simulink model "sensorless_MRAS_pmsm"  (Simulink 7.6)
settings: Solver=ode23tb  StartTime=0.0  StopTime=0.4  RelTol=1e-3
libraries: powerlib x11
settings Model: Creator=1  LastModifiedBy=1
settings OptimizationCC: InitFltsAndDblsToZero=on
settings DebuggingCC: SaveWithParameterizedLinksMsg=none  SignalResolutionControl=TryResolveAllWithWarning  MultiTaskDSMMsg=warning  MultiTaskCondExecSysMsg=none  UnconnectedLineMsg=none  StrictBusMsg=Warning
settings RTWCC: IncludeERTFirstTime=on
settings GRTTargetCC: TargetFcnLib=ansi_tfl_tmw.mat

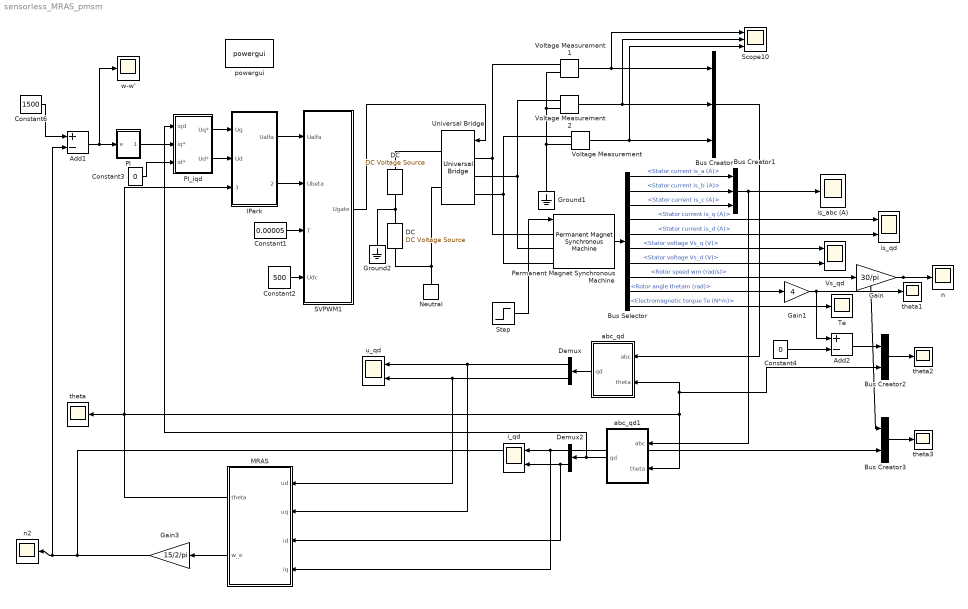
== system sensorless_MRAS_pmsm ==
  Add1 : Sum  Inputs=+-
  Add2 : Sum  Inputs=+-
  Bus Creator : BusCreator  Inputs=3
  Bus Creator1 : BusCreator  Inputs=3
  Bus Creator2 : BusCreator  Inputs=2
  Bus Creator3 : BusCreator  Inputs=2
  Bus Selector : BusSelector  OutputSignals=Stator current is_a (A),Stator current is_b (A),Stator current is_c (A),Stator current is_q (A),Stator current is_d (A),Stator voltage Vs_q (V),Stator voltage Vs_d (V),Rotor speed wm (rad/s),Rotor angle thetam (rad),Electromagnetic torque Te (N*m)
  Constant1 : Constant  Value=0.00005
  Constant2 : Constant  Value=500
  Constant3 : Constant  Value=0
  Constant4 : Constant  Value=0
  Constant6 : Constant  Value=1500
  DC : powerlib/Electrical Sources/DC Voltage Source  DialogController=POWERSYS.PowerSysDialog  SystemSampleTime=-1  Amplitude=250  Measurements=None
  "DC " : powerlib/Electrical Sources/DC Voltage Source  DialogController=POWERSYS.PowerSysDialog  SystemSampleTime=-1  Amplitude=250  Measurements=None
  Demux : Demux  Outputs=2
  Demux2 : Demux  Outputs=2
  Gain : Gain  Gain=30/pi
  Gain1 : Gain  Gain=4
  Gain3 : Gain  Gain=15/2/pi
  Ground1 : powerlib/Elements/Ground  DialogController=POWERSYS.PowerSysDialog  PhysicalDomain=powersysdomain  SubClassName=unknown  LeftPortType=p1  RightPortType=p1  LConnTagsString=a
  Ground2 : powerlib/Elements/Ground  DialogController=POWERSYS.PowerSysDialog  PhysicalDomain=powersysdomain  SubClassName=unknown  LeftPortType=p1  RightPortType=p1  LConnTagsString=a
  IPark : Subsystem
  MRAS : Subsystem
  Neutral : powerlib/Elements/Neutral  DialogController=POWERSYS.PowerSysDialog  PhysicalDomain=powersysdomain  SubClassName=unknown  LeftPortType=p1  RightPortType=p1  LConnTagsString=a  NodeNumber=10
  PI : Subsystem
  PI_iqd : Subsystem
  Permanent Magnet Synchronous Machine : powerlib/Machines/Permanent Magnet Synchronous Machine  DialogController=POWERSYS.PowerSysDialog  SystemSampleTime=-1  FluxDistribution=Sinusoidal  MechanicalLoad=Torque Tm  PresetModel=No  ShowDetailedParameters=on  Resistance=2.8750  Inductance=8.5e-3  dqInductances=[8.5e-3, 8.5e-3]  MachineConstant=Flux linkage established by magnets (V.s)  Flux=0.175  VoltageCst=126.966  TorqueCst=1.05  Flat=120  Mechanical="[ 1e-3, 0,  4 ]"  PolePairs=4  InitialConditions=[0,0, 0,0]  TsPowergui=0  TsBlock=-1
  SVPWM1 : Subsystem
  Scope10 : Scope  NumInputPorts=3
      settings: TimeRange=0.2  YMin=-250~-250~-250  YMax=250~250~250  SaveName=ScopeData22  DataFormat=Structure
  Step : Step  Time=0.2  SampleTime=0
  Te : Scope
      settings: YMin=1.775  YMax=2.225  SaveName=ScopeData6
  Universal Bridge : powerlib/Power Electronics/Universal Bridge  DialogController=POWERSYS.PowerSysDialog  SystemSampleTime=-1  Arms=3  SnubberResistance=1e5  SnubberCapacitance=inf  Device=IGBT / Diodes  Ron=1e-3  Lon=0  ForwardVoltages="[  0  0  ]"  ForwardVoltage=0  GTOparameters=[ 10e-6 , 20e-6 ]  IGBTparameters=[ 1e-6 , 2e-6 ]  Measurements=None  Measurements_2=None  converterType=Rectifier
  Voltage Measurement : powerlib/Measurements/Voltage Measurement  DialogController=POWERSYS.PowerSysDialog  SystemSampleTime=-1  PhasorSimulation=off  OutputType=Complex  PSBequivalent=0
  Voltage Measurement1 : powerlib/Measurements/Voltage Measurement  DialogController=POWERSYS.PowerSysDialog  SystemSampleTime=-1  PhasorSimulation=off  OutputType=Complex  PSBequivalent=0
  Voltage Measurement2 : powerlib/Measurements/Voltage Measurement  DialogController=POWERSYS.PowerSysDialog  SystemSampleTime=-1  PhasorSimulation=off  OutputType=Complex  PSBequivalent=0
  Vs_qd : Scope  NumInputPorts=2
      settings: TimeRange=0.4  YMin=-400~-99.99999999999994  YMax=400~-67.44186046511635  SaveName=ScopeData8
  abc_qd : Subsystem
  abc_qd1 : Subsystem
  "i_qd " : Scope  NumInputPorts=2
      settings: TimeRange=0.06  YMin=1.675~-0.475  YMax=2.075~-0.225  SaveName=ScopeData27  DataFormat=Structure
  is_abc (A) : Scope
      settings: TimeRange=0.06  YMin=-1.5  YMax=1.25  DataFormat=Structure
  is_qd : Scope  NumInputPorts=2
      settings: TimeRange=0.2  YMin=1.7~-0.23  YMax=2.1~-0.04  SaveName=ScopeData4
  n : Scope
      settings: TimeRange=0.0005809128630705485  YMin=2064.7  YMax=2065.35  SaveName=ScopeData15
  n2 : Scope
      settings: YMin=1470  YMax=1530  SaveName=ScopeData18
  powergui : powerlib/powergui  Priority=1  SystemSampleTime=-1  SimulationMode=Continuous  SampleTime=50e-6  frequency=60  SPID=off  DisableSnubberDevices=off  DisableRonSwitches=off  DisableVfSwitches=off  SwTol=0  Interpol=off  frequencyindice=0  echomessages=off  HookPort=off  DisplayEquations=off  FunctionMessages=off  EnableUseOfTLC=off  x0status=blocks  RestoreLinks=warning  ResistiveCurrentMeasurement=off  Ylog=off  Xlog=on  ShowGrid=off  save=off  variable=ZData  ZoomFFT=off  StartTime=0.0  cycles=1  DisplayStyle=1  FreqAxis=off  MaxFrequency=1000  frequencyindicesteady=1  display=off  methode=off
  theta{,1..3} (4 alike) : Scope
      theta settings: YMin=67.3  YMax=68.15  SaveName=ScopeData17
      theta1 settings: TimeRange=0.2  YMin=-3.955  YMax=-3.88  SaveName=ScopeData5
      theta2 settings: TimeRange=0.2  YMin=-10  YMax=55  SaveName=ScopeData7
      theta3 settings: TimeRange=0.2  YMin=-3.955  YMax=-3.88  SaveName=ScopeData14
  "u_qd " : Scope  NumInputPorts=2
      settings: TimeRange=0.06  YMin=-25~-250  YMax=325~350  SaveName=ScopeData26  DataFormat=Structure
  w-w' : Scope
      settings: TimeRange=0.02  YMin=-6  YMax=6  SaveName=ScopeData3
  wires:
  Constant3/1 -> PI_iqd/3(id*)
  Constant2/1 -> SVPWM1/4(Udc)
  Constant1/1 -> SVPWM1/3(T)
  Add1/1 -> PI/1(e), w-w'/1
  Constant6/1 -> Add1/1
  SVPWM1/1(Ugate) -> Universal Bridge/1
  IPark/1(Ualfa) -> SVPWM1/1(Ualfa)
  IPark/2(Ubeta) -> SVPWM1/2(Ubeta)
  Voltage Measurement/1 -> Scope10/3, Bus Creator/3
  Voltage Measurement2/1 -> Scope10/2, Bus Creator/2
  Voltage Measurement1/1 -> Scope10/1, Bus Creator/1
  Demux/1 -> "u_qd "/1, MRAS/2(uq)
  Demux/2 -> "u_qd "/2, MRAS/1(ud)
  Demux2/1 -> "i_qd "/1, MRAS/4(iq)
  Demux2/2 -> "i_qd "/2, MRAS/3(id)
  PI_iqd/2(Ud*) -> IPark/2(Ud)
  PI_iqd/1(Uq*) -> IPark/1(Uq)
  Permanent Magnet Synchronous Machine/1 -> Bus Selector/1
  Bus Selector/1 -> Bus Creator1/1  "<Stator current is_a (A)>"
  Bus Selector/2 -> Bus Creator1/2  "<Stator current is_b (A)>"
  Bus Selector/3 -> Bus Creator1/3  "<Stator current is_c (A)>"
  Bus Selector/4 -> is_qd/1  "<Stator current is_q (A)>"
  Bus Selector/5 -> is_qd/2  "<Stator current is_d (A)>"
  Bus Selector/6 -> Vs_qd/1  "<Stator voltage Vs_q (V)>"
  Bus Selector/7 -> Vs_qd/2  "<Stator voltage Vs_d (V)>"
  Gain/1 -> n/1, Bus Creator3/1
  Bus Selector/8 -> Gain/1  "<Rotor speed wm (rad/s)>"
  Bus Selector/9 -> Gain1/1  "<Rotor angle thetam (rad)>"
  Gain1/1 -> theta1/1, Add2/1
  Bus Selector/10 -> Te/1  "<Electromagnetic torque Te (N*m)>"
  Bus Creator1/1 -> is_abc (A)/1, abc_qd1/1(abc)
  Step/1 -> Permanent Magnet Synchronous Machine/1
  abc_qd/1(qd) -> Demux/1
  Gain3/1 -> n2/1, Add1/2, Bus Creator3/2
  abc_qd1/1(qd) -> Demux2/1, PI_iqd/1(iqd)
  MRAS/1(theta) -> IPark/3(thetma), abc_qd1/2(theta), abc_qd/2(theta), Bus Creator2/2, theta/1
  Bus Creator/1 -> abc_qd/1(abc)
  MRAS/2(w_e) -> Gain3/1
  PI/1(iq*) -> PI_iqd/2(iq*)
  Bus Creator2/1 -> theta2/1
  Bus Creator3/1 -> theta3/1
  Add2/1 -> Bus Creator2/1
  Constant4/1 -> Add2/2
  connections:
  Universal Bridge/RConn1 -- "DC "/RConn1
  DC/RConn1 -- "DC "/LConn1 -- Ground2/LConn1
  Voltage Measurement1/LConn2 -- Voltage Measurement2/LConn2 -- Ground1/LConn1 -- Voltage Measurement/LConn2
  DC/LConn1 -- Universal Bridge/RConn2 -- Neutral/LConn1
  Permanent Magnet Synchronous Machine/LConn1 -- Universal Bridge/LConn1 -- Voltage Measurement1/LConn1
  Permanent Magnet Synchronous Machine/LConn2 -- Universal Bridge/LConn2 -- Voltage Measurement2/LConn1
  Permanent Magnet Synchronous Machine/LConn3 -- Universal Bridge/LConn3 -- Voltage Measurement/LConn1

== system sensorless_MRAS_pmsm/IPark ==
  Uq : Inport
  Ud : Inport  Port=2
  thetma : Inport  Port=3
  Fcn : Fcn  Expr=cos(u[3])*u[2]-sin(u[3])*u[1]
  Fcn1 : Fcn  Expr=sin(u[3])*u[2]+cos(u[3])*u[1]
  Mux : Mux  Inputs=3
  Scope6 : Scope  NumInputPorts=2
      settings: YMin=40~20  YMax=230~220  SaveName=ScopeData12
  Ualfa : Outport
  Ubeta : Outport  Port=2
  wires:
  Uq/1 -> Mux/1
  Ud/1 -> Mux/2
  thetma/1 -> Mux/3
  Mux/1 -> Fcn/1, Fcn1/1
  Fcn/1 -> Ualfa/1, Scope6/1
  Fcn1/1 -> Ubeta/1, Scope6/2

== system sensorless_MRAS_pmsm/MRAS ==
  ud : Inport
  uq : Inport  Port=2
  id : Inport  Port=3
  iq : Inport  Port=4
  Integrator : Integrator
  Iqd : Subsystem
  "i_qd " : Scope  NumInputPorts=2
      settings: TimeRange=0.06  YMin=-4~0.5  YMax=16~10  SaveName=ScopeData23  DataFormat=Structure
  i_qd 1 : Scope  NumInputPorts=2
      settings: TimeRange=0.06  YMin=3.375~-1.525  YMax=3.8~-1.275  SaveName=ScopeData28  DataFormat=Structure
  we : Subsystem
  theta : Outport
  w_e : Outport  Port=2
  wires:
  ud/1 -> Iqd/1(ud)
  uq/1 -> Iqd/2(uq)
  iq/1 -> we/2(iq), "i_qd "/1
  Iqd/1(i_d) -> i_qd 1/2, we/3(i_d)
  Iqd/2(i_q) -> we/4(i_q), i_qd 1/1
  we/1(w_e) -> Integrator/1, w_e/1, Iqd/3(we)
  Integrator/1 -> theta/1
  id/1 -> we/1(id), "i_qd "/2

== system sensorless_MRAS_pmsm/PI ==
  e : Inport
  Integrator : Integrator
  Ks : Gain
  Ks/ts : Gain  Gain=0.02
  Saturation : Saturate  UpperLimit=21  LowerLimit=-21
  Sum1 : Sum  Inputs=|++
  iq* : Outport
  wires:
  Ks/1 -> Sum1/1
  Ks/ts/1 -> Integrator/1
  Integrator/1 -> Sum1/2
  e/1 -> Ks/1, Ks/ts/1
  Sum1/1 -> Saturation/1
  Saturation/1 -> iq*/1

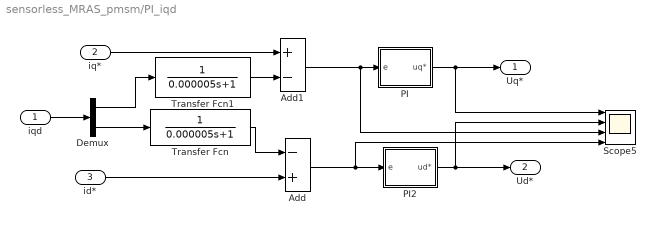
== system sensorless_MRAS_pmsm/PI_iqd ==
  iqd : Inport
  iq* : Inport  Port=2
  id* : Inport  Port=3
  Add : Sum  Inputs=-+
  Add1 : Sum  Inputs=+-
  Demux : Demux  Outputs=2
  PI : Subsystem
  PI2 : Subsystem
  Scope5 : Scope  NumInputPorts=4
      settings: YMin=218.5~-9.25~-0.2~-0.04  YMax=225~-7.75~0.25~0.06  SaveName=ScopeData10
  Transfer Fcn : TransferFcn  Denominator=[0.000005 1]
  Transfer Fcn1 : TransferFcn  Denominator=[0.000005 1]
  Uq* : Outport
  Ud* : Outport  Port=2
  wires:
  iqd/1 -> Demux/1
  id*/1 -> Add/2
  Add1/1 -> PI/1(e), Scope5/3
  Add/1 -> PI2/1(e), Scope5/4
  PI2/1(ud*) -> Ud*/1, Scope5/2
  PI/1(uq*) -> Uq*/1, Scope5/1
  Demux/1 -> Transfer Fcn1/1
  Transfer Fcn1/1 -> Add1/2
  Demux/2 -> Transfer Fcn/1
  Transfer Fcn/1 -> Add/1
  iq*/1 -> Add1/1

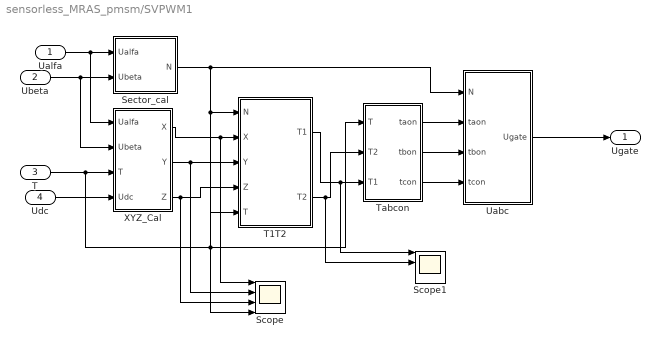
== system sensorless_MRAS_pmsm/SVPWM1 ==
  Ualfa : Inport
  Ubeta : Inport  Port=2
  T : Inport  Port=3
  Udc : Inport  Port=4
  Scope : Scope  NumInputPorts=4
      settings: YMin=0~-0.00015~1e-005~4.75  YMax=1.1e-020~-1e-005~0.00015~5.25  SaveName=ScopeData2
  Scope1 : Scope  NumInputPorts=4
      settings: YMin=3e-006~6.61744e-024~1e-005~4.75  YMax=1.6e-005~1e-007~0.00015~5.25  SaveName=ScopeData13
  Sector_cal : Subsystem
  T1T2 : Subsystem
  Tabcon : Subsystem
  Uabc : Subsystem
  XYZ_Cal : Subsystem
  Ugate : Outport
  wires:
  Sector_cal/1(N) -> Uabc/1(N), T1T2/1(N), Scope/4
  Ualfa/1 -> XYZ_Cal/1(Ualfa), Sector_cal/1(Ualfa)
  Ubeta/1 -> XYZ_Cal/2(Ubeta), Sector_cal/2(Ubeta)
  T/1 -> XYZ_Cal/3(T), Tabcon/1(T), T1T2/5(T)
  Udc/1 -> XYZ_Cal/4(Udc)
  XYZ_Cal/1(X) -> T1T2/2(X), Scope/1
  XYZ_Cal/2(Y) -> T1T2/3(Y), Scope/2
  XYZ_Cal/3(Z) -> T1T2/4(Z), Scope/3
  T1T2/2(T2) -> Tabcon/2(T2), Scope1/2
  T1T2/1(T1) -> Tabcon/3(T1), Scope1/1
  Tabcon/1(taon) -> Uabc/2(taon)
  Tabcon/2(tbon) -> Uabc/3(tbon)
  Tabcon/3(tcon) -> Uabc/4(tcon)
  Uabc/1(Ugate) -> Ugate/1

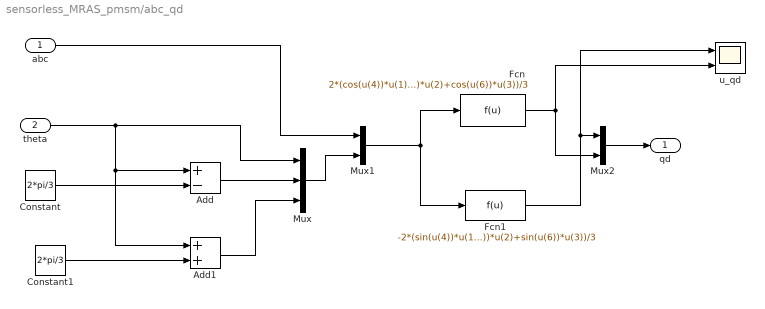
== system sensorless_MRAS_pmsm/abc_qd ==
  abc : Inport
  theta : Inport  Port=2
  Add : Sum  Inputs=+-
  Add1 : Sum
  Constant : Constant  Value=2*pi/3
  Constant1 : Constant  Value=2*pi/3
  Fcn : Fcn  Expr=2*(cos(u(4))*u(1)+cos(u(5))*u(2)+cos(u(6))*u(3))/3
  Fcn1 : Fcn  Expr=-2*(sin(u(4))*u(1)+sin(u(5))*u(2)+sin(u(6))*u(3))/3
  Mux : Mux  Inputs=3
  Mux1 : Mux  Inputs=2
  Mux2 : Mux  Inputs=2
  "u_qd " : Scope  NumInputPorts=2
      settings: TimeRange=0.06  YMin=-25~-300  YMax=300~250  SaveName=ScopeData24  DataFormat=Structure
  qd : Outport
  wires:
  Constant1/1 -> Add1/2
  Constant/1 -> Add/2
  theta/1 -> Mux/1, Add1/1, Add/1
  Add/1 -> Mux/2
  Add1/1 -> Mux/3
  Mux/1 -> Mux1/2
  abc/1 -> Mux1/1
  Mux1/1 -> Fcn/1, Fcn1/1
  Mux2/1 -> qd/1
  Fcn/1 -> Mux2/2, "u_qd "/2
  Fcn1/1 -> Mux2/1, "u_qd "/1

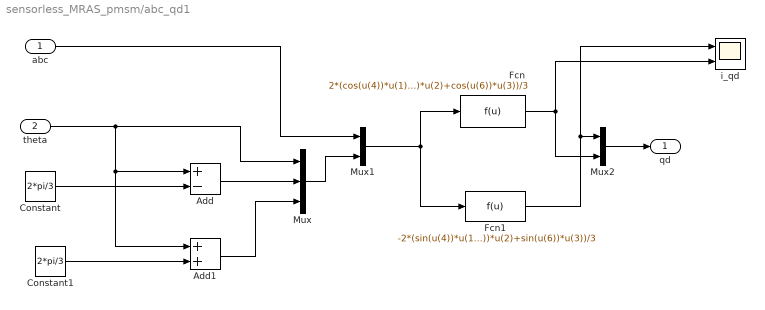
== system sensorless_MRAS_pmsm/abc_qd1 ==
  abc : Inport
  theta : Inport  Port=2
  Add : Sum  Inputs=+-
  Add1 : Sum
  Constant : Constant  Value=2*pi/3
  Constant1 : Constant  Value=2*pi/3
  Fcn : Fcn  Expr=2*(cos(u(4))*u(1)+cos(u(5))*u(2)+cos(u(6))*u(3))/3
  Fcn1 : Fcn  Expr=-2*(sin(u(4))*u(1)+sin(u(5))*u(2)+sin(u(6))*u(3))/3
  Mux : Mux  Inputs=3
  Mux1 : Mux  Inputs=2
  Mux2 : Mux  Inputs=2
  "i_qd " : Scope  NumInputPorts=2
      settings: TimeRange=0.06  YMin=-1~-4.25  YMax=2.5~-1  SaveName=ScopeData25  DataFormat=Structure
  qd : Outport
  wires:
  Constant1/1 -> Add1/2
  Constant/1 -> Add/2
  theta/1 -> Mux/1, Add1/1, Add/1
  Add/1 -> Mux/2
  Add1/1 -> Mux/3
  Mux/1 -> Mux1/2
  abc/1 -> Mux1/1
  Mux1/1 -> Fcn/1, Fcn1/1
  Mux2/1 -> qd/1
  Fcn/1 -> Mux2/2, "i_qd "/2
  Fcn1/1 -> Mux2/1, "i_qd "/1

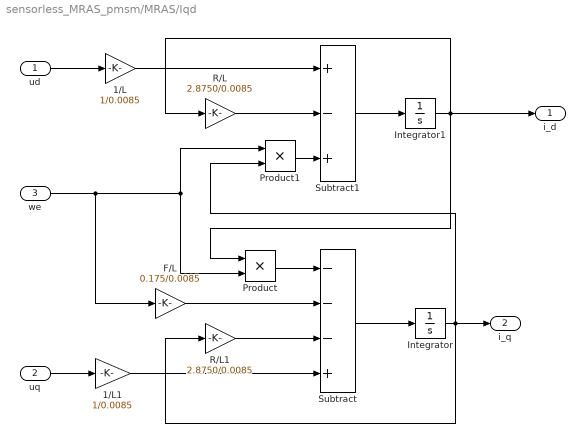
== system sensorless_MRAS_pmsm/MRAS/Iqd ==
  ud : Inport
  uq : Inport  Port=2
  we : Inport  Port=3
  1/L : Gain  Gain=1/0.0085
  1/L1 : Gain  Gain=1/0.0085
  F/L : Gain  Gain=0.175/0.0085
  Integrator : Integrator
  Integrator1 : Integrator
  Product : Product  RndMeth=Zero
  Product1 : Product  RndMeth=Zero
  R/L : Gain  Gain=2.8750/0.0085
  R/L1 : Gain  Gain=2.8750/0.0085
  Subtract : Sum  Inputs=---+
  Subtract1 : Sum  Inputs=+-+
  i_d : Outport
  i_q : Outport  Port=2
  wires:
  ud/1 -> 1/L/1
  uq/1 -> 1/L1/1
  1/L1/1 -> Subtract/4
  we/1 -> F/L/1, Product/2, Product1/1
  Subtract/1 -> Integrator/1
  Subtract1/1 -> Integrator1/1
  Integrator1/1 -> i_d/1, R/L/1, Product/1
  Integrator/1 -> i_q/1, Product1/2, R/L1/1
  1/L/1 -> Subtract1/1
  Product1/1 -> Subtract1/3
  R/L/1 -> Subtract1/2
  Product/1 -> Subtract/1
  F/L/1 -> Subtract/2
  R/L1/1 -> Subtract/3

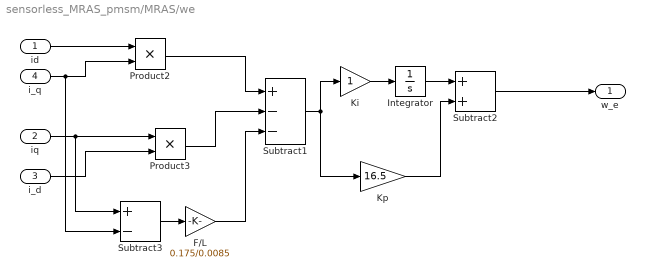
== system sensorless_MRAS_pmsm/MRAS/we ==
  id : Inport
  iq : Inport  Port=2
  i_d : Inport  Port=3
  i_q : Inport  Port=4
  F/L : Gain  Gain=0.175/0.0085
  Integrator : Integrator
  Ki : Gain
  Kp : Gain  Gain=16.5
  Product2 : Product  RndMeth=Zero
  Product3 : Product  RndMeth=Zero
  Subtract1 : Sum  Inputs=+--
  Subtract2 : Sum
  Subtract3 : Sum  Inputs=+-
  w_e : Outport
  wires:
  id/1 -> Product2/1
  i_q/1 -> Product2/2, Subtract3/2
  iq/1 -> Product3/1, Subtract3/1
  i_d/1 -> Product3/2
  Product2/1 -> Subtract1/1
  Product3/1 -> Subtract1/2
  Subtract3/1 -> F/L/1
  F/L/1 -> Subtract1/3
  Subtract1/1 -> Ki/1, Kp/1
  Ki/1 -> Integrator/1
  Integrator/1 -> Subtract2/1
  Subtract2/1 -> w_e/1
  Kp/1 -> Subtract2/2

== system sensorless_MRAS_pmsm/PI_iqd/PI ==
  e : Inport
  Integrator : Integrator
  Ki : Gain  Gain=15
  Ki/ti : Gain  Gain=2000
  Saturation : Saturate  UpperLimit=350  LowerLimit=-350
  Sum1 : Sum  Inputs=|++
  uq* : Outport
  wires:
  Ki/1 -> Sum1/1
  Ki/ti/1 -> Integrator/1
  Integrator/1 -> Sum1/2
  e/1 -> Ki/1, Ki/ti/1
  Sum1/1 -> Saturation/1
  Saturation/1 -> uq*/1

== system sensorless_MRAS_pmsm/PI_iqd/PI2 ==
  e : Inport
  Integrator : Integrator
  Ki : Gain  Gain=15
  Ki/ti : Gain  Gain=2000
  Saturation : Saturate  UpperLimit=50  LowerLimit=-50
  Sum1 : Sum  Inputs=|++
  ud* : Outport
  wires:
  Ki/1 -> Sum1/1
  Ki/ti/1 -> Integrator/1
  Integrator/1 -> Sum1/2
  Sum1/1 -> Saturation/1
  Saturation/1 -> ud*/1
  e/1 -> Ki/1, Ki/ti/1

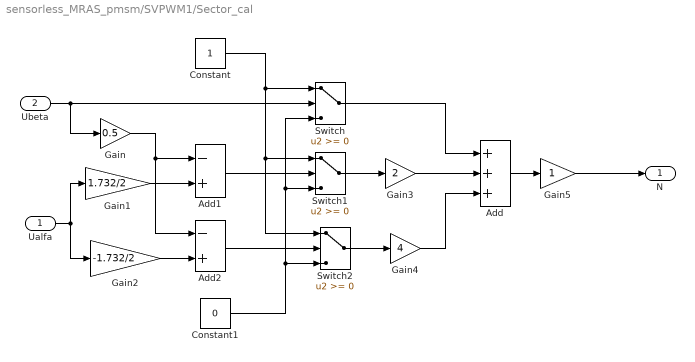
== system sensorless_MRAS_pmsm/SVPWM1/Sector_cal ==
  Ualfa : Inport
  Ubeta : Inport  Port=2
  Add : Sum  Inputs=+++
  Add1 : Sum  Inputs=-+
  Add2 : Sum  Inputs=-+
  Constant : Constant
  Constant1 : Constant  Value=0
  Gain : Gain  Gain=0.5
  Gain1 : Gain  Gain=1.732/2
  Gain2 : Gain  Gain=-1.732/2
  Gain3 : Gain  Gain=2
  Gain4 : Gain  Gain=4
  Gain5 : Gain  SampleTime=0.00005
  Switch : Switch
  Switch1 : Switch
  Switch2 : Switch
  N : Outport
  wires:
  Ubeta/1 -> Gain/1, Switch/2
  Ualfa/1 -> Gain2/1, Gain1/1
  Gain/1 -> Add1/1, Add2/1
  Gain1/1 -> Add1/2
  Gain2/1 -> Add2/2
  Add1/1 -> Switch1/2
  Add2/1 -> Switch2/2
  Switch1/1 -> Gain3/1
  Switch2/1 -> Gain4/1
  Switch/1 -> Add/1
  Gain3/1 -> Add/2
  Gain4/1 -> Add/3
  Constant/1 -> Switch/1, Switch1/1, Switch2/1
  Constant1/1 -> Switch1/3, Switch/3, Switch2/3
  Add/1 -> Gain5/1
  Gain5/1 -> N/1

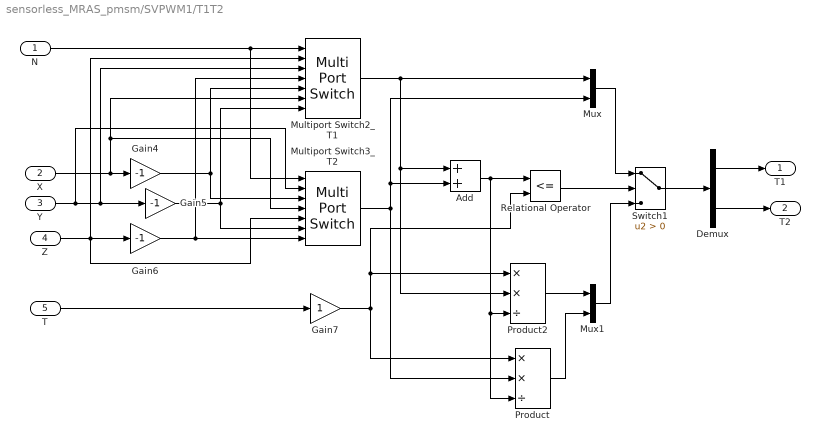
== system sensorless_MRAS_pmsm/SVPWM1/T1T2 ==
  N : Inport
  X : Inport  Port=2
  Y : Inport  Port=3
  Z : Inport  Port=4
  T : Inport  Port=5
  Add : Sum
  Demux : Demux  Outputs=2
  Gain4 : Gain  Gain=-1
  Gain5 : Gain  Gain=-1
  Gain6 : Gain  Gain=-1
  Gain7 : Gain
  Multiport Switch2_T1 : MultiPortSwitch  Inputs=6  zeroidx=off
  Multiport Switch3_T2 : MultiPortSwitch  Inputs=6  zeroidx=off
  Mux : Mux  Inputs=2
  Mux1 : Mux  Inputs=2
  Product : Product  Inputs=**/  RndMeth=Zero
  Product2 : Product  Inputs=**/  RndMeth=Zero
  Relational Operator : RelationalOperator  Operator=<=  OutDataTypeStr=boolean
  Switch1 : Switch  Criteria=u2 > Threshold
  T1 : Outport
  T2 : Outport  Port=2
  wires:
  N/1 -> Multiport Switch3_T2/1, Multiport Switch2_T1/1
  Y/1 -> Multiport Switch3_T2/2, Multiport Switch2_T1/3, Gain5/1
  X/1 -> Multiport Switch3_T2/4, Multiport Switch2_T1/6, Gain4/1
  Gain6/1 -> Multiport Switch2_T1/4, Multiport Switch3_T2/7
  Gain4/1 -> Multiport Switch2_T1/5, Multiport Switch3_T2/3
  Gain5/1 -> Multiport Switch2_T1/7, Multiport Switch3_T2/6
  Z/1 -> Gain6/1, Multiport Switch2_T1/2, Multiport Switch3_T2/5
  Multiport Switch2_T1/1 -> Mux/1, Add/1, Product2/2
  Multiport Switch3_T2/1 -> Add/2, Mux/2, Product/2
  Mux/1 -> Switch1/1
  Add/1 -> Relational Operator/1, Product2/3, Product/3
  Relational Operator/1 -> Switch1/2
  T/1 -> Gain7/1
  Gain7/1 -> Relational Operator/2, Product2/1, Product/1
  Product2/1 -> Mux1/1
  Product/1 -> Mux1/2
  Mux1/1 -> Switch1/3
  Switch1/1 -> Demux/1
  Demux/1 -> T1/1
  Demux/2 -> T2/1

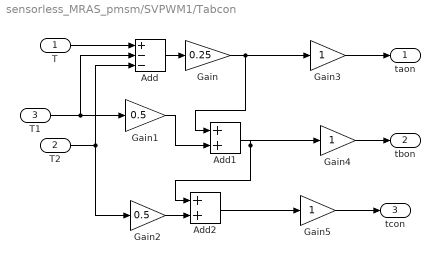
== system sensorless_MRAS_pmsm/SVPWM1/Tabcon ==
  T : Inport
  T2 : Inport  Port=2
  T1 : Inport  Port=3
  Add : Sum  Inputs=+--
  Add1 : Sum
  Add2 : Sum
  Gain : Gain  Gain=0.25
  Gain1 : Gain  Gain=0.5
  Gain2 : Gain  Gain=0.5
  Gain3 : Gain  SampleTime=0.00005
  Gain4 : Gain  SampleTime=0.00005
  Gain5 : Gain  SampleTime=0.00005
  taon : Outport
  tbon : Outport  Port=2
  tcon : Outport  Port=3
  wires:
  T2/1 -> Gain2/1, Add/3
  Add/1 -> Gain/1
  Gain/1 -> Add1/1, Gain3/1
  Gain1/1 -> Add1/2
  Add1/1 -> Add2/1, Gain4/1
  Gain2/1 -> Add2/2
  T/1 -> Add/1
  T1/1 -> Gain1/1, Add/2
  Gain5/1 -> tcon/1
  Add2/1 -> Gain5/1
  Gain4/1 -> tbon/1
  Gain3/1 -> taon/1

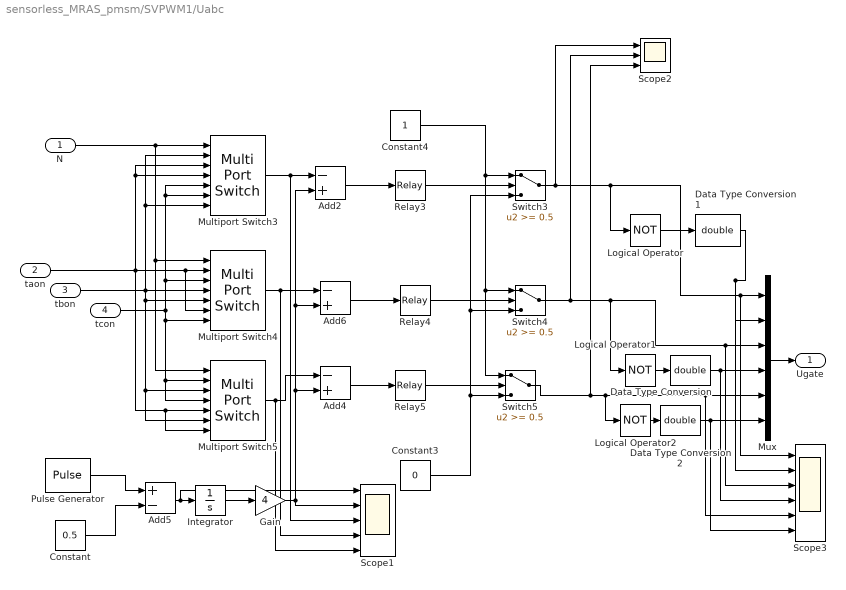
== system sensorless_MRAS_pmsm/SVPWM1/Uabc ==
  N : Inport
  taon : Inport  Port=2
  tbon : Inport  Port=3
  tcon : Inport  Port=4
  Add2 : Sum  Inputs=-+
  Add4 : Sum  Inputs=-+
  Add5 : Sum  Inputs=+-
  Add6 : Sum  Inputs=-+
  Constant : Constant  Value=0.5
  Constant3 : Constant  Value=0
  Constant4 : Constant
  Data Type Conversion : DataTypeConversion  OutDataTypeStr=double
  Data Type Conversion1 : DataTypeConversion  OutDataTypeStr=double
  Data Type Conversion2 : DataTypeConversion  OutDataTypeStr=double
  Gain : Gain  Gain=4
  Integrator : Integrator
  Logical Operator : Logic  Operator=NOT  AllPortsSameDT=off  OutDataTypeStr=boolean
  Logical Operator1 : Logic  Operator=NOT  AllPortsSameDT=off  OutDataTypeStr=boolean
  Logical Operator2 : Logic  Operator=NOT  AllPortsSameDT=off  OutDataTypeStr=boolean
  Multiport Switch3 : MultiPortSwitch  Inputs=6  zeroidx=off  SampleTime=0.00005
  Multiport Switch4 : MultiPortSwitch  Inputs=6  zeroidx=off  SampleTime=0.00005
  Multiport Switch5 : MultiPortSwitch  Inputs=6  zeroidx=off  SampleTime=0.00005
  Mux : Mux  Inputs=6
  Pulse Generator : DiscretePulseGenerator  PulseType=Time based  Period=0.00005  PulseWidth=50
  Relay3 : Relay  OnSwitchValue=0.0000002  OffSwitchValue=-0.0000002
  Relay4 : Relay  OnSwitchValue=0.0000002  OffSwitchValue=-0.0000002
  Relay5 : Relay  OnSwitchValue=0.0000002  OffSwitchValue=-0.0000002
  Scope1 : Scope  NumInputPorts=5
      settings: YMin=-0.5~-1e-005~-5e-006~-5e-006~-5e-006  YMax=0.5~6e-005~3e-005~3e-005~3e-005
  Scope2 : Scope  NumInputPorts=3
      settings: YMin=0~0~0  YMax=1~1~1  SaveName=ScopeData9  DataFormat=Structure
  Scope3 : Scope  NumInputPorts=6
      settings: YMin=0~0~0~0~0~0  YMax=1~1~1~1~1~1  SaveName=ScopeData11
  Switch3 : Switch  Threshold=0.5  ZeroCross=off
  Switch4 : Switch  Threshold=0.5  ZeroCross=off
  Switch5 : Switch  Threshold=0.5  ZeroCross=off
  Ugate : Outport
  wires:
  N/1 -> Multiport Switch5/1, Multiport Switch4/1, Multiport Switch3/1
  tbon/1 -> Multiport Switch5/6, Multiport Switch5/3, Multiport Switch4/5, Multiport Switch4/4, Multiport Switch3/7, Multiport Switch3/2
  taon/1 -> Multiport Switch5/7, Multiport Switch5/5, Multiport Switch4/6, Multiport Switch4/2, Multiport Switch3/4, Multiport Switch3/3
  tcon/1 -> Multiport Switch5/4, Multiport Switch5/2, Multiport Switch4/7, Multiport Switch4/3, Multiport Switch3/6, Multiport Switch3/5
  Multiport Switch3/1 -> Add2/1, Scope1/3
  Multiport Switch5/1 -> Add4/1, Scope1/5
  Add2/1 -> Relay3/1
  Add6/1 -> Relay4/1
  Add4/1 -> Relay5/1
  Relay3/1 -> Switch3/2
  Relay4/1 -> Switch4/2
  Relay5/1 -> Switch5/2
  Constant4/1 -> Switch3/1, Switch5/1, Switch4/1
  Constant3/1 -> Switch5/3, Switch3/3, Switch4/3
  Switch3/1 -> Logical Operator/1, Mux/1, Scope3/1, Scope2/1
  Switch4/1 -> Logical Operator1/1, Mux/3, Scope3/3, Scope2/2
  Switch5/1 -> Logical Operator2/1, Mux/5, Scope3/5, Scope2/3
  Multiport Switch4/1 -> Add6/1, Scope1/4
  Constant/1 -> Add5/2
  Add5/1 -> Integrator/1, Scope1/1
  Pulse Generator/1 -> Add5/1
  Integrator/1 -> Gain/1
  Gain/1 -> Add4/2, Add6/2, Add2/2, Scope1/2
  Mux/1 -> Ugate/1
  Logical Operator1/1 -> Data Type Conversion/1
  Data Type Conversion/1 -> Mux/4, Scope3/4
  Logical Operator/1 -> Data Type Conversion1/1
  Data Type Conversion1/1 -> Mux/2, Scope3/2
  Logical Operator2/1 -> Data Type Conversion2/1
  Data Type Conversion2/1 -> Mux/6, Scope3/6

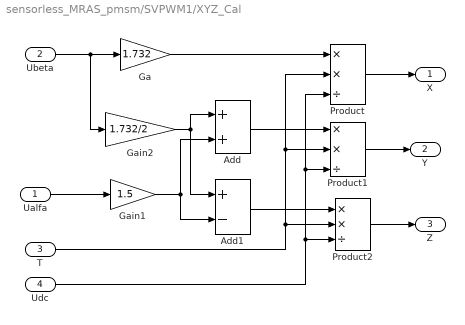
== system sensorless_MRAS_pmsm/SVPWM1/XYZ_Cal ==
  Ualfa : Inport
  Ubeta : Inport  Port=2
  T : Inport  Port=3
  Udc : Inport  Port=4
  Add : Sum
  Add1 : Sum  Inputs=+-
  Ga : Gain  Gain=1.732
  Gain1 : Gain  Gain=1.5
  Gain2 : Gain  Gain=1.732/2
  Product : Product  Inputs=**/  RndMeth=Zero
  Product1 : Product  Inputs=**/  RndMeth=Zero
  Product2 : Product  Inputs=**/  RndMeth=Zero
  X : Outport
  Y : Outport  Port=2
  Z : Outport  Port=3
  wires:
  Product/1 -> X/1
  Product1/1 -> Y/1
  Product2/1 -> Z/1
  Ubeta/1 -> Gain2/1, Ga/1
  Ga/1 -> Product/1
  T/1 -> Product2/2, Product1/2, Product/2
  Udc/1 -> Product2/3, Product1/3, Product/3
  Add/1 -> Product1/1
  Add1/1 -> Product2/1
  Gain2/1 -> Add/1, Add1/1
  Gain1/1 -> Add1/2, Add/2
  Ualfa/1 -> Gain1/1
